simulink model "AFM_SS_linearFDBK_obs_IMPLEMENT_outer_integral_track"  (R2016b)
settings: Solver=VariableStepDiscrete  StartTime=0.0  StopTime=trun  FixedStep=Ts  EnableMultiTasking=on
undefined symbols (not defined in the file): absorbDelay, K, Ki, L, NoiseP, PLANT, sys_obs, Ts, umax, x0_int, x0_obs
libraries: simulink x1, cstblocks x1
settings Model: Creator=arnold  LastModifiedBy=arnold
settings DataIOCC: SaveFormat=Structure  SaveOutput=off  SaveState=on  InspectSignalLogs=on  TimeSaveName=tout_ptos
settings OptimizationCC: LifeSpan=inf
settings DebuggingCC: SolverPrmCheckMsg=warning  SFUnexpectedBacktrackingDiag=warning  SFNoUnconditionalDefaultTransitionDiag=warning  SFExecutionAtInitializationDiag=none
settings HardwareCC: ProdBitPerPointer=32  ProdBitPerSizeT=32  ProdBitPerPtrDiffT=32  ProdLargestAtomicFloat=None  ProdIntDivRoundTo=Undefined  ProdEndianess=Unspecified  ProdWordSize=32  ProdHWDeviceType=32-bit Generic
settings ModelReferenceCC: PropagateSignalLabelsOutOfModel=off
settings GRTTargetCC: TargetLangStandard=C89/C90 (ANSI)  GeneratePreprocessorConditionals=Disable all
settings ConfigComp: CovMetricSettings=dw  CovHtmlReporting=on  CovSaveCumulativeToWorkspaceVar=on  CovSaveSingleToWorkspaceVar=on  CovExternalEMLEnable=off  CovSFcnEnable=off

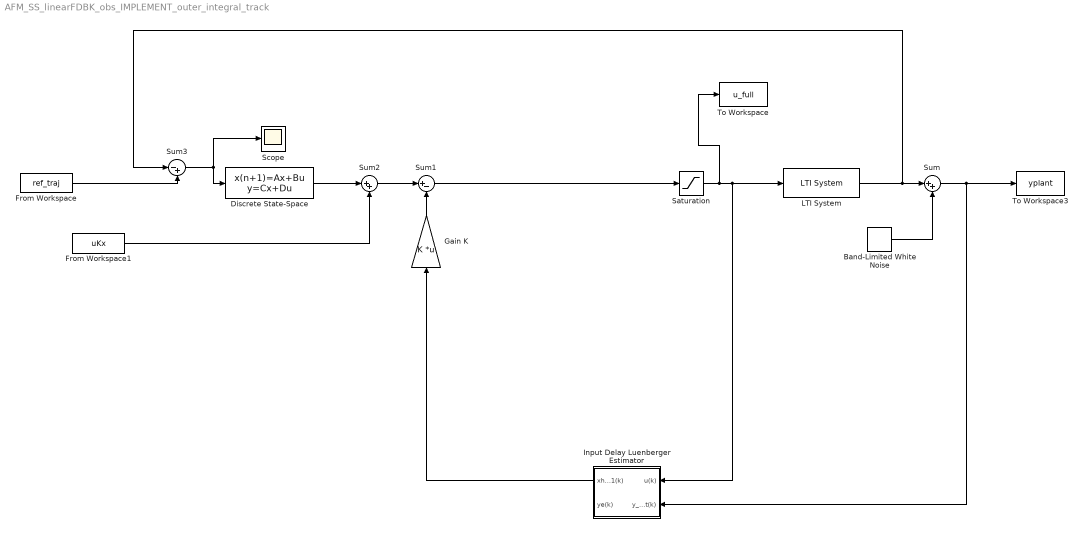
== system AFM_SS_linearFDBK_obs_IMPLEMENT_outer_integral_track ==
  Band-Limited White Noise : simulink/Sources/Band-Limited White Noise  Cov=[NoiseP]  Ts=Ts  seed=[23341]
  Discrete State-Space : DiscreteStateSpace  B=Ki  D=0  X0=x0_int  SampleTime=Ts
  From Workspace : FromWorkspace  VariableName=ref_traj  SampleTime=Ts
  From Workspace1 : FromWorkspace  VariableName=uKx  SampleTime=Ts
  Gain K : Gain  Gain=K  Multiplication=Matrix(K*u)
  Input Delay Luenberger Estimator : Subsystem  AncestorBlock=customLibFcns/Input Delay Luenberger Estimator
  LTI System : cstblocks/LTI System  sys=absorbDelay(PLANT)  IC=x0_full
  Saturation : Saturate  UpperLimit=umax  LowerLimit=-umax
  Scope : Scope
  Sum : Sum  Inputs=|++
  Sum1 : Sum  Inputs=|+-
  Sum2 : Sum  Inputs=|++
  Sum3 : Sum  Inputs=|-+
  To Workspace : ToWorkspace  VariableName=u_full  SaveFormat=Timeseries  SampleTime=-1
      settings: Save2DSignal=2-D array (concatenate along first dimension)
  To Workspace3 : ToWorkspace  VariableName=yplant  SaveFormat=Timeseries  SampleTime=-1
      settings: Save2DSignal=2-D array (concatenate along first dimension)
  wires:
  LTI System/1 -> Sum/1, Sum3/1
  Gain K/1 -> Sum1/2
  Input Delay Luenberger Estimator/1(xhat_1(k)) -> Gain K/1
  From Workspace/1 -> Sum3/2
  Sum3/1 -> Discrete State-Space/1, Scope/1
  From Workspace1/1 -> Sum2/2
  Sum/1 -> Input Delay Luenberger Estimator/2(y_plant(k)), To Workspace3/1
  Band-Limited White Noise/1 -> Sum/2
  Saturation/1 -> To Workspace/1, Input Delay Luenberger Estimator/1(u(k)), LTI System/1
  Sum1/1 -> Saturation/1
  Discrete State-Space/1 -> Sum2/1
  Sum2/1 -> Sum1/1

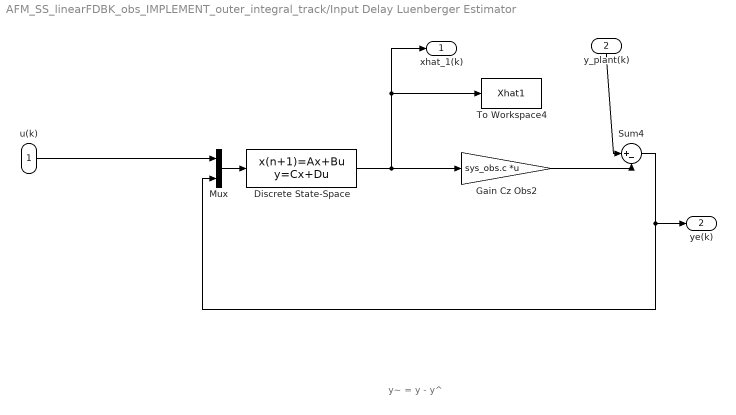
== system AFM_SS_linearFDBK_obs_IMPLEMENT_outer_integral_track/Input Delay Luenberger Estimator ==
  note: y~ = y - y^
  u(k) : Inport
  y_plant(k) : Inport  Port=2
  Discrete State-Space : DiscreteStateSpace  A=sys_obs.a  B=[sys_obs.b, L]  C=eye(length(sys_obs.b))  D=zeros(length(sys_obs.b), 2)  X0=x0_obs  SampleTime=Ts
  Gain Cz Obs2 : Gain  Gain=sys_obs.c  Multiplication=Matrix(K*u)
  Mux : Mux  Inputs=2
  Sum4 : Sum  Inputs=|+-
  To Workspace4 : ToWorkspace  VariableName=Xhat1  SaveFormat=Timeseries  SampleTime=-1
      settings: Save2DSignal=2-D array (concatenate along first dimension)
  xhat_1(k) : Outport
  ye(k) : Outport  Port=2
  wires:
  Sum4/1 -> ye(k)/1, Mux/2
  u(k)/1 -> Mux/1
  Mux/1 -> Discrete State-Space/1
  Discrete State-Space/1 -> Gain Cz Obs2/1, To Workspace4/1, xhat_1(k)/1
  Gain Cz Obs2/1 -> Sum4/2
  y_plant(k)/1 -> Sum4/1
